simulink model "test"  (R2019a)
settings: Solver=ode1  StartTime=0.0  StopTime=5e-3  FixedStep=50e-6  RelTol=1e-3
libraries: powerlib x13, powerlib_meascontrol x2
settings Model: Creator=abruyere  LastModifiedBy=abruyere

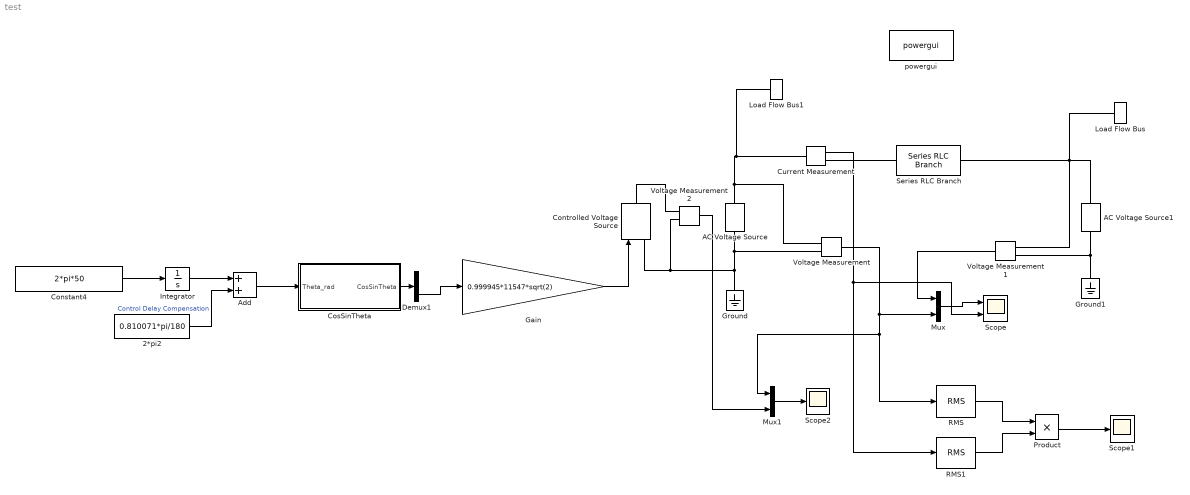
== system test ==
  2*pi2 : Constant  Value=0.810071*pi/180
  AC Voltage Source : powerlib/Electrical Sources/AC Voltage Source  Amplitude=0.999945*11547*sqrt(2)  Phase=0.810071  Frequency=50  SampleTime=0  Measurements=None  BusType=PQ  Pref=50000  Qref=0  Qmin=-inf  Qmax=+inf
      settings: SourceProductName=Simscape Electrical
  AC Voltage Source1 : powerlib/Electrical Sources/AC Voltage Source  Amplitude=1*11547*sqrt(2)  Phase=0  Frequency=50  SampleTime=0  Measurements=None  BusType=swing  Pref=1000  Qref=500  Qmin=-inf  Qmax=+inf
      settings: SourceProductName=Simscape Electrical
  Add : Sum
  Constant4 : Constant  Value=2*pi*50
  Controlled Voltage Source : powerlib/Electrical Sources/Controlled Voltage Source  Initialize=on  Source_Type=AC  Amplitude=0  Phase=0  Frequency=0  Measurements=None
      settings: SourceProductName=Simscape Electrical
  CosSinTheta : Subsystem
  Current Measurement : powerlib/Measurements/Current Measurement  PhasorSimulation=off  OutputType=Complex  PSBequivalent=0
      settings: SourceProductName=Simscape Electrical
  Demux1 : Demux  Outputs=2
  Gain : Gain  Gain=0.999945*11547*sqrt(2)
  Ground : powerlib/Elements/Ground  LConnTagsString=a
      settings: SourceProductName=Simscape Electrical
  Ground1 : powerlib/Elements/Ground  LConnTagsString=a
      settings: SourceProductName=Simscape Electrical
  Integrator : Integrator
  Load Flow Bus : powerlib/Measurements/Load Flow Bus  LConnTagsString=a  Phases=A  Connectors=on one side  ID=BUS01  Vbase=20e3/sqrt(3)  Vref=1  Vangle=0  VLF=1  VLFb=NaN  VLFc=NaN  angleLF=0  angleLFb=NaN  angleLFc=NaN
      settings: SourceProductName=Simscape Electrical
  Load Flow Bus1 : powerlib/Measurements/Load Flow Bus  LConnTagsString=a  Phases=A  Connectors=on one side  ID=BUS02  Vbase=20e3/sqrt(3)  Vref=1  Vangle=0  VLF=0.9999  VLFb=NaN  VLFc=NaN  angleLF=0.8101  angleLFb=NaN  angleLFc=NaN
      settings: SourceProductName=Simscape Electrical
  Mux : Mux  Inputs=2
  Mux1 : Mux  Inputs=2
  Product : Product
  RMS : powerlib_meascontrol/Measurements/RMS  TrueRMS=on  Freq=50  RMSInit=120  Ts=0
      settings: SourceProductName=Simscape Electrical
  RMS1 : powerlib_meascontrol/Measurements/RMS  TrueRMS=on  Freq=50  RMSInit=120  Ts=0
      settings: SourceProductName=Simscape Electrical
  Scope : Scope  NumInputPorts=2
  Scope1 : Scope
  Scope2 : Scope
  Series RLC Branch : powerlib/Elements/Series RLC Branch  LConnTagsString=__new0  RConnTagsString=__new0  BranchType=RL  Resistance=0.12  Inductance=120e-3  SetiL0=off  InitialCurrent=0  Capacitance=1e-6  Setx0=off  InitialVoltage=0  Measurements=None
      settings: SourceProductName=Simscape Electrical
  Voltage Measurement : powerlib/Measurements/Voltage Measurement  PhasorSimulation=off  OutputType=Complex  PSBequivalent=0
      settings: SourceProductName=Simscape Electrical
  Voltage Measurement1 : powerlib/Measurements/Voltage Measurement  PhasorSimulation=off  OutputType=Complex  PSBequivalent=0
      settings: SourceProductName=Simscape Electrical
  Voltage Measurement2 : powerlib/Measurements/Voltage Measurement  PhasorSimulation=off  OutputType=Complex  PSBequivalent=0
      settings: SourceProductName=Simscape Electrical
  powergui : powerlib/powergui  Priority=1  SimulationMode=Discrete  SampleTime=50e-6  frequency=60  Iterations=150  frequencyindice=50  Pbase=1e6  ErrMax=1e-05  UnitsV=V  UnitsW=W  buscounter=0  FunctionMessages=off  echomessages=off  EnableUseOfTLC=off  CurrentSourceSwitches=off  DisableSnubberDevices=off  DisableRonSwitches=off  DisableVfSwitches=off  DisplayEquations=off  AutomaticDiscreteSolvers=off  SolverType=Tustin/Backward Euler (TBE)  Interpol=off  ExternalGateDelay=off  methode=off  Ts=100  x0status=steady  SPID=on  SwTol=0  HookPort=off  NonlinearTolerance=0  nMaxIteration=15  ContinueOnMaxIteration=off  RestoreLinks=warning  ResistiveCurrentMeasurement=off  Frange=[0:2:500]  Ylog=off  Xlog=on  ShowGrid=off  save=off  variable=ZData  structure=0  ZoomFFT=off  StartTime=0.0  cycles=1  DisplayStyle=1  fundamental=60  FreqAxis=off  MaxFrequency=1000  frequencyindicesteady=1  RmsSteady=1  display=off
      settings: SourceProductName=Simscape Electrical
  wires:
  Voltage Measurement1/1 -> Mux/1
  Voltage Measurement/1 -> Mux1/1, RMS/1, Mux/2
  Mux/1 -> Scope/1
  Current Measurement/1 -> RMS1/1, Scope/2
  RMS/1 -> Product/1
  RMS1/1 -> Product/2
  Product/1 -> Scope1/1
  Constant4/1 -> Integrator/1
  Add/1 -> CosSinTheta/1(Theta_rad)
  Integrator/1 -> Add/1
  CosSinTheta/1(CosSinTheta) -> Demux1/1
  Demux1/2 -> Gain/1
  Gain/1 -> Controlled Voltage Source/1
  2*pi2/1 -> Add/2  "Control Delay Compensation"
  Voltage Measurement2/1 -> Mux1/2
  Mux1/1 -> Scope2/1
  connections:
  AC Voltage Source/LConn1 -- Voltage Measurement2/LConn2 -- Controlled Voltage Source/LConn1 -- Ground/LConn1 -- Voltage Measurement/LConn2
  Series RLC Branch/RConn1 -- Load Flow Bus/LConn1 -- Voltage Measurement1/LConn1 -- AC Voltage Source1/RConn1
  Ground1/LConn1 -- AC Voltage Source1/LConn1 -- Voltage Measurement1/LConn2
  Current Measurement/RConn1 -- Series RLC Branch/LConn1
  AC Voltage Source/RConn1 -- Voltage Measurement/LConn1 -- Load Flow Bus1/LConn1 -- Current Measurement/LConn1
  Controlled Voltage Source/RConn1 -- Voltage Measurement2/LConn1

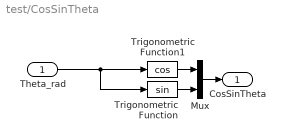
== system test/CosSinTheta ==
  Theta_rad : Inport
  Mux : Mux  Inputs=2
  Trigonometric Function : Trigonometry
  Trigonometric Function1 : Trigonometry  Operator=cos
  CosSinTheta : Outport
  wires:
  Theta_rad/1 -> Trigonometric Function/1, Trigonometric Function1/1
  Trigonometric Function/1 -> Mux/2
  Mux/1 -> CosSinTheta/1
  Trigonometric Function1/1 -> Mux/1
